simulink model "regulator_LQR_discrete_comparison_Ueq"  (Simulink 10.0)
settings: Solver=ode45  StartTime=0.0  StopTime=tsim  RelTol=1e-3  EnableMultiTasking=on
values from neighbouring files (symbols this model uses):
  C_states = eye(2)    [es3.m]
  D_states = [0 0]'    [es3.m]
  Klqr1 = dlqr(A,B,Q,R)    [es3.m]
  sat_max = inf    [es3.m]
  sat_min = -inf    [es3.m]
  Ts = 0.1    [es3.m]
  Ubar = inv(dcgain(Gz))*Ybar    [es3.m]
  x0 = [5 20]    [es3.m]
  xref = Xbar    [es3.m]
undefined symbols (not defined in the file or in its folder): A, B, C, Klqr2
settings Model: Creator=Administrator  LastModifiedBy=Chiara
settings DataIOCC: LimitDataPoints=on  SignalLoggingSaveFormat=ModelDataLogs
settings OptimizationCC: ExpressionDepthLimit=2147483647  InitFltsAndDblsToZero=on
settings DebuggingCC: SolverPrmCheckMsg=warning  FcnCallInpInsideContextMsg=warning  StateNameClashWarn=warning
settings GRTTargetCC: GeneratePreprocessorConditionals=Disable all
settings ConfigComp: CovExternalEMLEnable=off  CovSFcnEnable=off

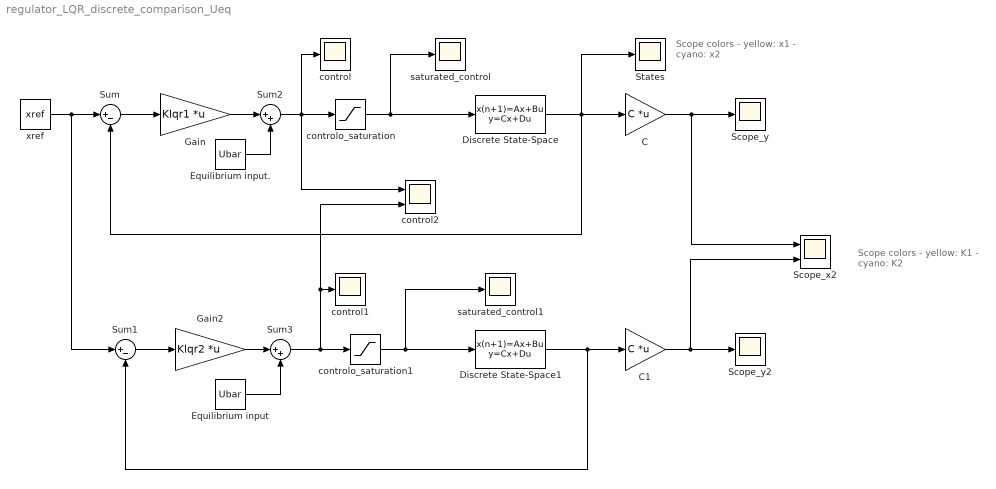
== system regulator_LQR_discrete_comparison_Ueq ==
  note: Scope colors
      | - yellow: x1
      | - cyano: x2
  note: Scope colors
      | - yellow: K1
      | - cyano: K2
  C : Gain  Gain=C  Multiplication=Matrix(K*u)
  C1 : Gain  Gain=C  Multiplication=Matrix(K*u)
  Discrete State-Space : DiscreteStateSpace  A=A  B=B  C=C_states  D=D_states  InitialCondition=x0  SampleTime=Ts
  Discrete State-Space1 : DiscreteStateSpace  A=A  B=B  C=C_states  D=D_states  InitialCondition=x0  SampleTime=Ts
  "Equilibrium input " : Constant  Value=Ubar
  "Equilibrium input. " : Constant  Value=Ubar
  Gain : Gain  Gain=Klqr1  Multiplication=Matrix(K*u)
  Gain2 : Gain  Gain=Klqr2  Multiplication=Matrix(K*u)
  Scope_x2 : Scope  NumInputPorts=2
  Scope_y : Scope
  Scope_y2 : Scope
  States : Scope
  Sum : Sum  Inputs=|+-
  Sum1 : Sum  Inputs=|+-
  Sum2 : Sum  Inputs=|++
  Sum3 : Sum  Inputs=|++
  control : Scope
  control1 : Scope
  control2 : Scope  NumInputPorts=2
  controlo_saturation : Saturate  UpperLimit=sat_max  LowerLimit=sat_min
  controlo_saturation1 : Saturate  UpperLimit=sat_max  LowerLimit=sat_min
  saturated_control : Scope
  saturated_control1 : Scope
  xref : Constant  Value=xref
  wires:
  controlo_saturation/1 -> Discrete State-Space/1, saturated_control/1
  Sum/1 -> Gain/1
  Discrete State-Space/1 -> States/1, C/1, Sum/2
  Discrete State-Space1/1 -> C1/1, Sum1/2
  Sum1/1 -> Gain2/1
  controlo_saturation1/1 -> Discrete State-Space1/1, saturated_control1/1
  xref/1 -> Sum1/1, Sum/1
  C/1 -> Scope_x2/1, Scope_y/1
  C1/1 -> Scope_x2/2, Scope_y2/1
  Gain/1 -> Sum2/1
  Sum2/1 -> control2/1, control/1, controlo_saturation/1
  "Equilibrium input. "/1 -> Sum2/2
  Gain2/1 -> Sum3/1
  Sum3/1 -> controlo_saturation1/1, control2/2, control1/1
  "Equilibrium input "/1 -> Sum3/2
